simulink model "Electrode"  (R2024b)
settings: Solver=ode1  StartTime=0.0  StopTime=10.0  FixedStep=0.0005  RelTol=1e-3
settings Model: Creator=wai484  LastModifiedBy=wai484
settings SolverCC: EnableFixedStepZeroCrossing=on
settings DataIOCC: SaveOutput=off  SaveTime=off
settings ModelReferenceCC: ModelReferenceMinAlgLoopOccurrences=on
settings GRTTargetCC: CombineOutputUpdateFcns=off

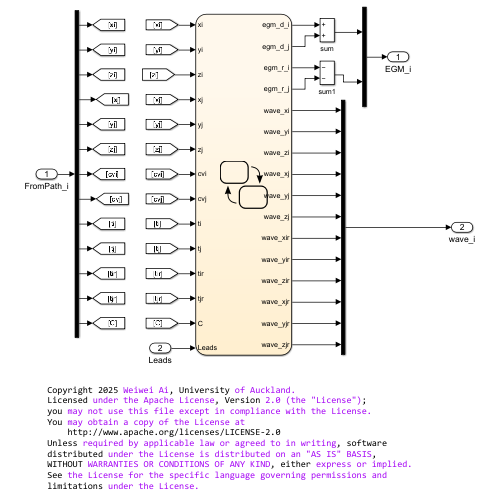
[thumbnail: Simulink's stored preview of the top-level diagram]
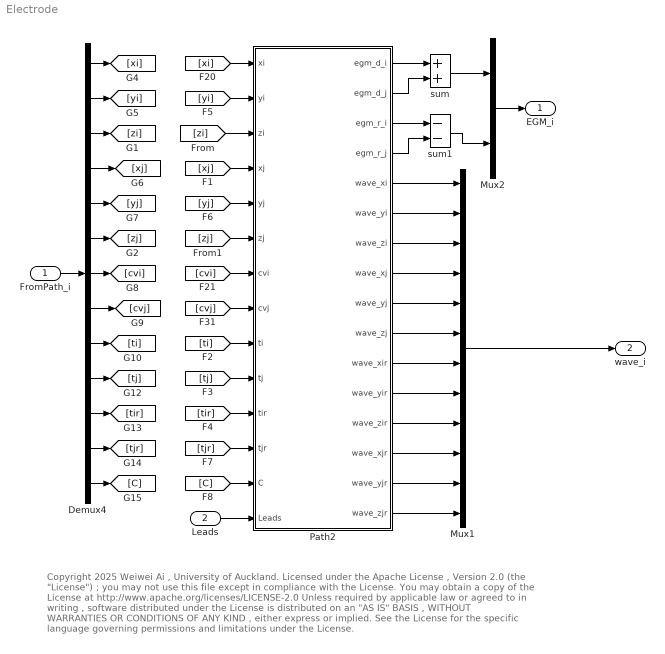
== system Electrode ==
  note: Copyright 2025 Weiwei Ai , University of Auckland.
      | Licensed under the Apache License , Version 2.0 (the "License") ;
      | you may not use this file except in compliance with the License.
      | You may obtain a copy of the License at
      | http://www.apache.org/licenses/LICENSE-2.0
      | Unless required by applicable law or agreed to in writing , software
      | distributed under the License is distributed on an "AS IS" BASIS ,
      | WITHOUT WARRANTIES OR CONDITIONS OF ANY KIND , either express or implied.
      | See the License for the specific language governing permissions and
      | limitations under the License.
  FromPath_i : Inport  OutDataTypeStr=double  PortDimensions=13
  Leads : Inport  Port=2  OutDataTypeStr=double  PortDimensions=28
  Demux4 : Demux  Outputs=13
  Mux1 : Mux  Inputs=12
  Mux2 : Mux  Inputs=2
  Path2 : Stateflow chart  TreatAsAtomicUnit=on
  sum : Sum
  sum1 : Sum  Inputs=--
  EGM_i : Outport  OutDataTypeStr=double  PortDimensions=[1 8]  SampleTime=[0.00050000000000000001,0]
  wave_i : Outport  Port=2  OutDataTypeStr=double  PortDimensions=12  SampleTime=[0.00050000000000000001,0]
  wires:
  Mux2/1 -> EGM_i/1
  [xi] -> Path2/1(xi)
  [xj] -> Path2/4(xj)
  [yi] -> Path2/2(yi)
  [yj] -> Path2/5(yj)
  [cvi] -> Path2/7(cvi)
  [cvj] -> Path2/8(cvj)
  FromPath_i/1 -> Demux4/1
  Demux4/1 -> [xi]
  Demux4/2 -> [yi]
  [C] -> Path2/13(C)
  [tjr] -> Path2/12(tjr)
  [tir] -> Path2/11(tir)
  [tj] -> Path2/10(tj)
  [ti] -> Path2/9(ti)
  Leads/1 -> Path2/14(Leads)
  Mux1/1 -> wave_i/1
  sum/1 -> Mux2/1
  Path2/1(egm_d_i) -> sum/1
  Path2/2(egm_d_j) -> sum/2
  sum1/1 -> Mux2/2
  Path2/3(egm_r_i) -> sum1/1
  Path2/4(egm_r_j) -> sum1/2
  Demux4/13 -> [C]
  Demux4/12 -> [tjr]
  Demux4/11 -> [tir]
  Demux4/10 -> [tj]
  Demux4/9 -> [ti]
  Demux4/8 -> [cvj]
  Demux4/7 -> [cvi]
  Demux4/5 -> [yj]
  Demux4/4 -> [xj]
  Demux4/3 -> [zi]
  Demux4/6 -> [zj]
  [zi] -> Path2/3(zi)
  [zj] -> Path2/6(zj)
  Path2/5(wave_xi) -> Mux1/1
  Path2/6(wave_yi) -> Mux1/2
  Path2/7(wave_zi) -> Mux1/3
  Path2/8(wave_xj) -> Mux1/4
  Path2/9(wave_yj) -> Mux1/5
  Path2/10(wave_zj) -> Mux1/6
  Path2/11(wave_xir) -> Mux1/7
  Path2/12(wave_yir) -> Mux1/8
  Path2/13(wave_zir) -> Mux1/9
  Path2/14(wave_xjr) -> Mux1/10
  Path2/15(wave_yjr) -> Mux1/11
  Path2/16(wave_zjr) -> Mux1/12

== stateflow chart Electrode/Path2 ==
  state EGM1
    state De_wave_i [parallel]
      settings: executionOrder=1
      state Idle
        en:
        egm_d_i=[0 0 0 0]; wave_xi=0; wave_yi=0; wave_zi=0;
      state Active
        du:
        [egm_d_i,wave_xi,wave_yi,wave_zi]  = EGM(cvi,xi,yi,zi,xj,yj,zj,ti,Leads,C);
      EGM1.De_wave_i.Idle -> EGM1.De_wave_i.Active : [ti~=0]
      (default) -> EGM1.De_wave_i.Idle
      EGM1.De_wave_i.Active -> EGM1.De_wave_i.Idle : [ti==0]
    state De_wave_j [parallel]
      settings: executionOrder=2
      state Idle
        en:
        egm_d_j=[0 0 0 0]; wave_xj=0; wave_yj=0; wave_zj=0;
      state Active
        du:
        [egm_d_j,wave_xj,wave_yj, wave_zj]  = EGM(cvj,xj,yj,zj,xi,yi,zi,tj,Leads,C);
      EGM1.De_wave_j.Idle -> EGM1.De_wave_j.Active : [tj~=0]
      (default) -> EGM1.De_wave_j.Idle
      EGM1.De_wave_j.Active -> EGM1.De_wave_j.Idle : [tj==0]
    state Re_wave_i [parallel]
      settings: executionOrder=3
      state Idle
        en:
        egm_r_i=[0 0 0 0]; wave_xir=0; wave_yir=0; wave_zir=0;
      state Active
        du:
        [egm_r_i,wave_xir,wave_yir, wave_zir]  = EGM(cvi,xi,yi,zi,xj,yj,zj,tir,Leads,C);
      EGM1.Re_wave_i.Idle -> EGM1.Re_wave_i.Active : [tir~=0]
      (default) -> EGM1.Re_wave_i.Idle
      EGM1.Re_wave_i.Active -> EGM1.Re_wave_i.Idle : [tir==0]
    state Re_wave_j [parallel]
      settings: executionOrder=4
      state Active
        du:
        [egm_r_j,wave_xjr,wave_yjr, wave_zjr]  = EGM(cvj,xj,yj,zj,xi,yi,zi,tjr,Leads,C);
      state Idle
        en:
        egm_r_j=[0 0 0 0]; wave_xjr=0; wave_yjr=0; wave_zjr=0;
      EGM1.Re_wave_j.Idle -> EGM1.Re_wave_j.Active : [tjr~=0]
      (default) -> EGM1.Re_wave_j.Idle
      EGM1.Re_wave_j.Active -> EGM1.Re_wave_j.Idle : [tjr==0]
  (default) -> EGM1
  data: cv1in function_input; x1in function_input; y1in function_input; z1in function_input; x2in function_input; y2in function_input; z2in function_input; t1in function_input; electrodein function_input; Cin function_input; Potential_d function_output; x11 function_output; y11 function_output; z11 function_output; xi input; yi input; zi input; xj input; yj input; zj input; cvi input; cvj input; ti input; tj input; tir input; tjr input; C input; egm_d_i output; egm_d_j output; egm_r_i output; egm_r_j output; wave_xi output; wave_yi output; wave_zi output; wave_xj output; wave_yj output; wave_zj output; Leads input; wave_xir output; wave_yir output; wave_zir output; wave_xjr output; wave_yjr output; wave_zjr output
  function [Potential_d,x11,y11,z11]  = EGM(cv1in,x1in,y1in,z1in,x2in,y2in,z2in,t1in,electrodein,Cin):
    | function [Potential_d,x11,y11,z11]  = EGM(cv1in,x1in,y1in,z1in,x2in,y2in,z2in,t1in,electrodein,Cin)
    | %#codegen
    | % ==============================================================
    | %  3D Discrete Moving Dipole Model (Longitudinal + Transversal)
    | %
    | %  The dipole moves from r1 = (x1,y1,z1) to r2 = (x2,y2,z2)
    | %  with speed cv1in.
    | %
    | %  The sensed potential at electrode location r_p is:
    | %
    | %      V = L_scale * (p_long · R)/|R|^3  +  T_scale * (p_trans · R)/|R|^3
    | %
    | %  where:
    | %      D̂     = longitudinal dipole direction (direction of propagation)
    | %      n⊥     = transversal dipole direction (unit vector ⟂ to D̂)
    | %      R      = vector from dipole to electrode
    | %      |R|    = distance from dipole to electrode
    | %
    | % ==============================================================
    | 
    | %% ---------------- Dipole trajectory -------------------------
    | r1 = [x1in, y1in, z1in];
    | r2 = [x2in, y2in, z2in];
    | 
    | D  = r2 - r1;        % displacement vector
    | L  = norm(D);        % path length
    | % if path has zero length, handle gracefully (no motion, dipole fixed at r1)
    | if L == 0
    |     D_hat = [0 0 0]; % Longitudinal dipole (unit vector along motion)
    |     s = 0;
    |     rd = r1;
    | else
    |     D_hat = D / L; % Longitudinal dipole (unit vector along motion)
    |     % dipole position at time t1
    |     s = cv1in * t1in / L;     % fractional position
    |     s = min(max(s,0),1);      % clamp
    |     rd = r1 + s * D;          % dipole coordinates at time t1
    | end
    | 
    | x11 = rd(1);
    | y11 = rd(2);
    | z11 = rd(3);
    | 
    | %% ------------- Electrode group counts ------------------------
    | vtip = electrodein(end);
    | vring = electrodein(end-1);
    | atip = electrodein(end-2);
    | aring = electrodein(end-3);
    | 
    | % total number of electrodes = (vtip+vring+atip+aring)
    | N = (vtip + vring + atip + aring) * 3;
    | 
    | Potential_d  = zeros(1,4);
    | p = zeros(1, N/3);
    | 
    | %% ------------------ Dipole vectors ----------------------------
    | 
    | 
    | % --- choose a transversal direction perpendicular to D_hat
    | % We need any vector n_perp such that n_perp · D_hat = 0 and ||n_perp|| = 1
    | if L == 0
    |     % choose arbitrary orthonormal basis
    |     n_perp = [0 0 1];
    | else
    |     % pick a temp vector not parallel to D_hat:
    |     if abs(D_hat(1)) < 0.9
    |         temp = [1 0 0];
    |     else
    |         temp = [0 1 0];
    |     end
    |     n_perp = cross(D_hat, temp);
    |     n_perp_norm = norm(n_perp);
    |     if n_perp_norm < 1e-12
    |         % fallback (very rare): try different temp
    |         temp = [0 0 1];
    |         n_perp = cross(D_hat, temp);
    |         n_perp_norm = norm(n_perp);
    |         if n_perp_norm < 1e-12
    |             % give up and set default
    |             n_perp = [0 0 1];
    |         else
    |             n_perp = n_perp / n_perp_norm;
    |         end
    |     else
    |         n_perp = n_perp / n_perp_norm;
    |     end
    | end
    | 
    | % final longitudinal and transversal dipole directions
    | p_long  = D_hat;
    | p_trans = n_perp;
    | 
    | % weighting of longitudinal and transversal terms
    | L_scale = 1.0;
    | T_scale = 0.1;
    | %% ------------- Loop through all microelectrodes ---------------
    | m = 0;
    | % small regularizer to avoid infinite values when r==0
    | r_eps = 1e-9 * max(1, L);
    | for j = 1:3:(N-2)
    | 
    |     % electrode location
    |     x3 = electrodein(j);
    |     y3 = electrodein(j+1);
    |     z3 = electrodein(j+2);
    |     rp = [x3, y3, z3];
    | 
    |     % vector from dipole to electrode
    |     R = rp - rd;
    |     r = norm(R);
    |     if r < r_eps
    |         r = r_eps;
    |     end
    |     % ----------- Longitudinal dipole potential -----------------
    |     %
    |     %    V_long = (p_long · R) / |R|^3
    |     % -----------------------------------------------------------
    |     V_long = L_scale * dot(p_long, R) / (r^3);
    | 
    |     % ----------- Transversal dipole potential ------------------
    |     %
    |     %    V_trans = (p_trans · R) / |R|^3
    |     %
    |     %   (represents curvature / spread normal to propagation)
    |     % -----------------------------------------------------------
    |     V_trans = T_scale * dot(p_trans, R) / (r^3);
    | 
    |     % Total potential at this microelectrode
    |     EGMall = V_long + V_trans;
    |     m = m + 1;
    |     p(m) = EGMall * Cin;
    | end
    | s=1;
    | e=aring;
    | Potential_d(1)=sum(p(s:e));
    | s=e+1;
    | e=s+atip-1;
    | Potential_d(2)=sum(p(s:e));
    | s=e+1;
    | e=s+vring-1;
    | Potential_d(3)=sum(p(s:e));
    | s=e+1;
    | e=s+vtip-1;
    | Potential_d(4)=sum(p(s:e));
    | 
    | end
